simulink model "master_thesis_simulink"  (R2022a)
settings: Solver=VariableStepAuto  StartTime=0.0  StopTime=p_0p.time(end)  FixedStep=0.001  RelTol=1e-3
values from neighbouring files (symbols this model uses):
  markers_forearm = [0.00210510253906 -0.143263397217 -0.00798474121094]    [markers_forearm.mat]
  markers_shoulder = [0.010127746582 -0.151647644043 -0.0119686279297]    [markers_shoulder.mat]
undefined symbols (not defined in the file or in its folder): arm, DiscIntNeverNeededParam, Discrete, ekf, kf, LS, m, markers_hand, n, noise, q0, q0_LS, q0_model, sample_Time, selected, state_observer, Time, tSh_0_0Conf, X, Y, Z
libraries: sm_lib x2029, nesl_utility x1553, robotlib x75, ctrlSharedLib x8
(part 68 of 70)

== matlab function master_thesis_simulink/Ros2Matlab/S1_F0_H3/Position_M0 & velocity_M0 computation/MATLAB Function3 ==
  data: M0_isNew input; y output; M1_isNew input; M2_isNew input; M3_isNew input; M4_isNew input
 function y = fcn(M0_isNew, M1_isNew, M2_isNew, M3_isNew, M4_isNew)

if (M0_isNew == 0 || M1_isNew == 0 || M2_isNew == 0 || M3_isNew == 0 || M4_isNew == 0)
%if (M0_isNew == 0 || M1_isNew == 0 || M2_isNew == 0)

    y = -1;

else

    y = 1;
end

== matlab function master_thesis_simulink/Ros2Matlab/S1_F0_H3/tSh_0 computation/If Action Subsystem1/Mi_M0_POS1 ==
  data: p0_W input; pSh_W input; quat_02W input; tSh_0 output
function tSh_0  = fcn(p0_W, pSh_W, quat_02W)

% p_0 and v_0 are wrt M0_RF
% p_Sh wrt Sh_RF
% p_Fo wrt Fo_RF
% p_Wr wrt Wr_RF

% Number of markers
%m = size(p_W, 1) / 3;

%% Position/velocity of the markers wrt M0
tSh_0 = zeros(3, 1);

%% Quaternion describing rotation of M0 wrt W
quat_02W = reshape(quat_02W(1:4), [1, 4]);

%R =Rz*Ry*Rx;

%% Rotation: 0 to W
R_02W = quat2rotm(quat_02W);


tSh_0 = -R_02W'*p0_W + R_02W'*pSh_W;

== matlab function master_thesis_simulink/Ros2Matlab/S1_F0_H3/tSh_0 computation/MATLAB Function3 ==
  data: M0_isNew input; y output; Sh_isNew input
function y = fcn(M0_isNew, Sh_isNew)

if (M0_isNew == 0 || Sh_isNew == 0)

    y = -1;

else

    y = 1;
end

== matlab function master_thesis_simulink/Experiments/S1_F0_H3/Experiments/EKF/Extended Kalman Filter ==
  settings: updateMethod=DISCRETE
  data: p_0p input; v_0p input; shoulder_variables input; forearm_variables input; hand_variables input; qk output; Pk output; ekf parameter; noise parameter
function [qk, Pk] = KF(p_0p, v_0p, shoulder_variables, forearm_variables, hand_variables, ekf, noise)

% Extended Kalman filter algorithm 
% The following EKF algorithm estimate the state qk based on :
% -- The previous estimate qk_1 
% -- The input v_0 at time k
% -- The measurement p_0 at time k

% Inputs:
% -- p_0        : Measurement at time k
% -- v_0        : Input at time k

% Output:
% -- qk         : EKF estimate 
% -- Pk         : Covariance matrix of the state

%% Extrinsic functions
coder.extrinsic('f_f_mex');
coder.extrinsic('f_Phi_mex');
coder.extrinsic('f_Fekf_mex');
coder.extrinsic('f_Gekf_mex');
coder.extrinsic('f_Hekf_mex');
coder.extrinsic('eigs');

%% Define flags to understand if there are any markers in SHOULDER, FOREARM, HAND
flag_sh = shoulder_variables;
flag_fo = forearm_variables;
flag_ha = hand_variables;

if (shoulder_variables == -1)

    flag_sh = [];
end

if (forearm_variables == -1)

    flag_fo = [];
end

if (hand_variables == -1)

    flag_ha = [];
end

%% Number of markers
m = size(p_0p, 1) / 3;

%% Number of DoF
n = size(ekf.q0, 1);

%% Initialization

% Fk initialization
Fk = zeros(n, n);

% Gk initialization
Gk = zeros(n, m*3);

% Hk initialization
Hk = zeros(m*3, n);

% Phi_qk_ initialization
Phi_qk_ = zeros(m*3, 1);

% qk_ initialization
qk_ = zeros(n, 1);

%% Current state estimate, covariance
persistent qk_1 Pk_1;

if isempty(qk_1)

    %% %% First iteration
    qk = ekf.q0;
    qk_1 = qk;
    Pk = ekf.P0;
    Pk_1 = Pk;

else
   
    %% %% Next iterations

    %% Process Noise 
    % Gk computation
    Gk = full(f_Gekf_mex(qk_1, flag_sh, flag_fo, flag_ha, v_0p));

    % Q
%     noise.Q = Gk * noise.Rv * Gk'* 100;
%     noise.Q = (noise.Q + noise.Q') / 2; 
%     
%     % Check if Q is a Covariance matrix
%     is_Symmetric = issymmetric(noise.Q);
%     is_PosDef = false;
%     if ~is_Symmetric
% 
%         disp('Q not Symmetric');
%     else
%         
%         eig = zeros(n, 1);
%         eig = eigs(noise.Q, n);
%         if all(eig > 0)
%             is_PosDef = true;
%         end
%     end
% 
%     if ~is_PosDef
% 
%         disp('Q not Positve Definite');       
%     end
    
    %% TIME update
    % Predicted state
    qk_ = full(f_f_mex(qk_1, flag_sh, flag_fo, flag_ha, v_0p));

    % Fk computation
    Fk = full(f_Fekf_mex(qk_1, flag_sh, flag_fo, flag_ha, v_0p));

    % Predicted Covariance
    Pk_ = Fk * Pk_1 * Fk' + noise.Q;
    
    %% MEASUREMENT update
    % Hk computation
    Hk = full(f_Hekf_mex(qk_, flag_sh, flag_fo, flag_ha));

    % Kalman Gain 
    Kk = Pk_ * Hk' / (Hk * Pk_ * Hk' + noise.R);

    % Phi(qk_)
    Phi_qk_ = full(f_Phi_mex(qk_, flag_sh, flag_fo, flag_ha));

    % Updated state
    qk = wrapToPi(qk_ + Kk * (p_0p - Phi_qk_));
    qk_1 = qk;

    % Updated Covariance
    Pk = (eye(n) - Kk * Hk) * Pk_ * (eye(n) - Kk * Hk)' + Kk * noise.R * Kk';
    Pk_1 = Pk;

end
end

== matlab function master_thesis_simulink/Experiments/S1_F0_H3/Experiments/EKF/p_0p - Phi(q_EKF) ==
  data: p_0p input; q_EKF input; error_FK output; shoulder_variables input; forearm_variables input; hand_variables input
function error_FK  = FK(p_0p, q_EKF, shoulder_variables, forearm_variables, hand_variables)

% Computes the joints' velocities (LEAST SQUARES)

% Inputs:
% -- q                     : current joint variables configuration
% -- u                     : markers' velocities measurements
% -- shoulder_variables    : matrix containing markers position wrt SHOULDER Base RF
% -- forearm_variables     : matrix containing markers position wrt FOREARM Base RF
% -- hand_variables        : matrix containing markers position wrt HAND Base RF


% Output:
% -- Phi                   : Position of the markers wrt World RF
% -- J                     : Jacobian evaluated at the current joints variables estimate

% Extrinsic functions
coder.extrinsic('f_Phi_mex');
 
% Define flags to understand if there are any markers in SHOULDER, FOREARM, HAND
flag_sh = shoulder_variables;
flag_fo = forearm_variables;
flag_ha = hand_variables;

if (shoulder_variables == -1)

    flag_sh = [];
end

if (forearm_variables == -1)

    flag_fo = [];
end

if (hand_variables == -1)

    flag_ha = [];
end

% Initialization
p_FK = zeros(12, 1);

% Phi(q_EKF)
p_FK = full(f_Phi_mex(q_EKF, flag_sh, flag_fo, flag_ha));

% p_0 - Phi(q_EKF)
error_FK = p_0p - p_FK;

== matlab function master_thesis_simulink/Experiments/S1_F0_H3/Experiments/Human arm/MATLAB Function2 ==
  data: shoulder input; y output
function y = fcn(shoulder)

y = shoulder(1:3, :);

== matlab function master_thesis_simulink/Experiments/S1_F0_H3/Experiments/Human arm/MATLAB Function3 ==
  data: forearm input; y output
function y = fcn(forearm)

y = forearm(1:3, :);

== matlab function master_thesis_simulink/Experiments/S1_F0_H3/Experiments/Human arm/MATLAB Function4 ==
  data: hand input; y output size=[3 2]
function y = fcn(hand)

y = hand(1:3, :);

== matlab function master_thesis_simulink/Experiments/S1_F0_H3/Experiments/KF/Kalman Filter ==
  data: Delta_pk input; Delta_uk input; Delta_qk output; kf parameter; Pk output; noise parameter; p00 input
function [Delta_qk, Pk] = KF(Delta_pk, Delta_uk, kf, noise, p00)

% Kalman filter algorithm 
% The following KF algorithm estimate the quantity Delta_qk based on :
% -- The previous estimate xk_1 
% -- The input u_eqk at time k
% -- The measurement Delta_pk at time k

% Inputs:
% -- Delta_pk       : Measurement at time k
% -- Delta_uk       : Input at time k

% Output:
% -- Delta_qk       : KF estimate 
% -- Pk             : Covariance matrix of the state

persistent iteration;
% Previous state estimate
persistent Delta_qk_1 Pk_1;

persistent Delta_pk_1 Delta_uk_1

% Number of markers
m = size(kf.H, 1) / 3;
% Number of DoF
n = size(kf.F, 1);

% qk_ initialization
Delta_qk_ = zeros(n, 1);

% qk initialization
Delta_qk = zeros(n, 1);

% Pk initialization
Pk = zeros(n, n);

% Initialization
% if isempty(iteration)
% 
%     iteration = 1;
%     Delta_qk_1 = kf.Delta_q0;
%     Delta_qk = Delta_qk_1;
%     Pk = kf.Pk(1:n, 1:n);
%     iteration = iteration + 1;
% 
% else
% 
%     % Prediction ste
%     Delta_qk_ = kf.F * Delta_qk_1 + kf.G * u_eq;
%     
%     % Update step
%     Delta_qk = Delta_qk_ + kf.Kk(1:n, 3*m*(iteration-2)+1:3*m*(iteration-2)+3*m) * (Delta_pk - kf.H * Delta_qk_);
% 
%     if (iteration < 10)
% 
%         disp(abs(Delta_qk - Delta_qk_1))
%     end
%     Delta_qk_1 = Delta_qk;
%     Pk = kf.Pk(1:n, n*(iteration-1)+1:n*(iteration-1)+n);
%     iteration = iteration + 1;
% end

if isempty(Delta_qk_1)

    iteration = 1;

 
    % MEASUREMENT update
    Kk = p00 * kf.H' / (kf.H * p00 * kf.H' + noise.R);
    Delta_qk = Kk * (Delta_pk - kf.H*kf.Delta_q0);
    Delta_qk_1 = Delta_qk;
    Pk = p00;
    Pk_1 = Pk;
else
    
    % TIME update
    Delta_qk_ = kf.F*Delta_qk_1 + kf.G*Delta_uk;
    Pk_ = kf.F * Pk_1 * kf.F' + noise.Q;
    
    % MEASUREMENT update
    Kk = Pk_ * kf.H' / (kf.H * Pk_ * kf.H' + noise.R);
    Delta_qk = Delta_qk_ + Kk * (Delta_pk - kf.H*Delta_qk_);
    
    Delta_qk_1 = Delta_qk;
    Pk = (eye(n) - Kk * kf.H) * Pk_ * (eye(n) - Kk * kf.H)' + Kk * noise.R * Kk';
    Pk_1 = Pk;
    
    if (iteration == 2)
    
        disp('KF ')
        disp(Kk);
    end
end

iteration = iteration + 1;
end

== matlab function master_thesis_simulink/Experiments/S1_F0_H3/Experiments/KF/MATLAB Function ==
  data: n_k output; noise parameter
function n_k = fcn(noise)

% Generate a sample from normal distribution with covariance matrix N
coder.extrinsic('mvnrnd');

% Number of markers 
m = size(noise.N, 1) / 3;

% Initialization
n_k = zeros(m*3, 1);

n_k = mvnrnd(zeros(m*3, 1), noise.N, 1)';

== matlab function master_thesis_simulink/Experiments/S1_F0_H3/Experiments/KF/trial/Kalman Filter ==
  data: Delta_pk input; Delta_uk input; Delta_qk output; kf parameter; Pk output
function [Delta_qk, Pk] = KF(Delta_pk, Delta_uk, kf)

% Kalman filter algorithm 
% The following KF algorithm estimate the quantity Delta_qk based on :
% -- The previous estimate xk_1 
% -- The input u_eqk at time k
% -- The measurement Delta_pk at time k

% Inputs:
% -- Delta_pk       : Measurement at time k
% -- Delta_uk       : Input at time k

% Output:
% -- Delta_qk       : KF estimate 
% -- Pk             : Covariance matrix of the state

persistent iteration;
% Previous state estimate
persistent Delta_qk_1;

% Number of markers
m = size(kf.H, 1) / 3;
% Number of DoF
n = size(kf.F, 1);

% Initialization
if isempty(iteration)

    iteration = 1;
    Delta_qk_1 = kf.x0est;
    Delta_qk = Delta_qk_1;
    Pk = kf.Pk(1:n, 1:n);
    iteration = iteration + 1;

else

    % Prediction step
    Delta_qk_ = kf.F * Delta_qk_1 - kf.G * Delta_uk;
    
    % Update step
    Delta_qk = Delta_qk_ + kf.Kk(1:n, 3*m*(iteration-2)+1:3*m*(iteration-2)+3*m) * (Delta_pk - kf.H * Delta_qk_);
    Delta_qk_1 = Delta_qk;
    Pk = kf.Pk(1:n, n*(iteration-1)+1:n*(iteration-1)+n);
    iteration = iteration + 1;
end

== matlab function master_thesis_simulink/Experiments/S1_F1_H2/Experiments/EKF/Extended Kalman Filter ==
  settings: updateMethod=DISCRETE
  data: p_0p input; v_0p input; shoulder_variables input; forearm_variables input; hand_variables input; qk output; Pk output; ekf parameter; noise parameter
function [qk, Pk] = KF(p_0p, v_0p, shoulder_variables, forearm_variables, hand_variables, ekf, noise)

% Extended Kalman filter algorithm 
% The following EKF algorithm estimate the state qk based on :
% -- The previous estimate qk_1 
% -- The input v_0 at time k
% -- The measurement p_0 at time k

% Inputs:
% -- p_0        : Measurement at time k
% -- v_0        : Input at time k

% Output:
% -- qk         : EKF estimate 
% -- Pk         : Covariance matrix of the state

%% Extrinsic functions
coder.extrinsic('f_f_mex');
coder.extrinsic('f_Phi_mex');
coder.extrinsic('f_Fekf_mex');
coder.extrinsic('f_Gekf_mex');
coder.extrinsic('f_Hekf_mex');
coder.extrinsic('eigs');

%% Define flags to understand if there are any markers in SHOULDER, FOREARM, HAND
flag_sh = shoulder_variables;
flag_fo = forearm_variables;
flag_ha = hand_variables;

if (shoulder_variables == -1)

    flag_sh = [];
end

if (forearm_variables == -1)

    flag_fo = [];
end

if (hand_variables == -1)

    flag_ha = [];
end

%% Number of markers
m = size(p_0p, 1) / 3;

%% Number of DoF
n = size(ekf.q0, 1);

%% Initialization

% Fk initialization
Fk = zeros(n, n);

% Gk initialization
Gk = zeros(n, m*3);

% Hk initialization
Hk = zeros(m*3, n);

% Phi_qk_ initialization
Phi_qk_ = zeros(m*3, 1);

% qk_ initialization
qk_ = zeros(n, 1);

%% Current state estimate, covariance
persistent qk_1 Pk_1;

if isempty(qk_1)

    %% %% First iteration
    qk = ekf.q0;
    qk_1 = qk;
    Pk = ekf.P0;
    Pk_1 = Pk;

else
   
    %% %% Next iterations

    %% Process Noise 
    % Gk computation
    Gk = full(f_Gekf_mex(qk_1, flag_sh, flag_fo, flag_ha, v_0p));

    % Q
%     noise.Q = Gk * noise.Rv * Gk'* 100;
%     noise.Q = (noise.Q + noise.Q') / 2; 
%     
%     % Check if Q is a Covariance matrix
%     is_Symmetric = issymmetric(noise.Q);
%     is_PosDef = false;
%     if ~is_Symmetric
% 
%         disp('Q not Symmetric');
%     else
%         
%         eig = zeros(n, 1);
%         eig = eigs(noise.Q, n);
%         if all(eig > 0)
%             is_PosDef = true;
%         end
%     end
% 
%     if ~is_PosDef
% 
%         disp('Q not Positve Definite');       
%     end
    
    %% TIME update
    % Predicted state
    qk_ = full(f_f_mex(qk_1, flag_sh, flag_fo, flag_ha, v_0p));

    % Fk computation
    Fk = full(f_Fekf_mex(qk_1, flag_sh, flag_fo, flag_ha, v_0p));

    % Predicted Covariance
    Pk_ = Fk * Pk_1 * Fk' + noise.Q;
    
    %% MEASUREMENT update
    % Hk computation
    Hk = full(f_Hekf_mex(qk_, flag_sh, flag_fo, flag_ha));

    % Kalman Gain 
    Kk = Pk_ * Hk' / (Hk * Pk_ * Hk' + noise.R);

    % Phi(qk_)
    Phi_qk_ = full(f_Phi_mex(qk_, flag_sh, flag_fo, flag_ha));

    % Updated state
    qk = wrapToPi(qk_ + Kk * (p_0p - Phi_qk_));
    qk_1 = qk;

    % Updated Covariance
    Pk = (eye(n) - Kk * Hk) * Pk_ * (eye(n) - Kk * Hk)' + Kk * noise.R * Kk';
    Pk_1 = Pk;

end
end

== matlab function master_thesis_simulink/Experiments/S1_F0_H3/Experiments/KF/trial/Linearized Discrete Model ==
  data: Delta_uk input; Delta_qk output; Delta_pk output; kf parameter
function [Delta_qk, Delta_pk] = LDM(Delta_uk, kf)

% Discrete model linearized around the equilibrium point [q_eq, u_eq]

% This function computes both the outputs (markers' position) and the
% states (joints' variables) without considering the measurement noise

% Delta_qk+1 = F*Delta_qk + G*Delta_uk
% Delta_pk = H*Delta_qk

% Input:
% -- Delta_uk       : Delta_uk = uk - u_eqk at time k

% Output:
% -- Delta_qk       : States at time k
% -- Delta_pk       : outputs at time k

% Previous state
persistent Delta_qk_1; 

if isempty(Delta_qk_1)

    % Initial condition
    Delta_qk_1 = kf.q0 - kf.equilibrium_q;
    Delta_qk = Delta_qk_1;

else

    % State equation
    Delta_qk = kf.F * Delta_qk_1 + kf.G * Delta_uk;
    Delta_qk_1 = Delta_qk;

end

% Output equation
Delta_pk = kf.H * Delta_qk;

== matlab function master_thesis_simulink/Experiments/S1_F0_H3/Experiments/LS/LS ==
  data: q input; v_0 input; qdot_LS output; shoulder_variables input; forearm_variables input; hand_variables input
function qdot_LS  = LS(q, v_0, shoulder_variables, forearm_variables, hand_variables)

% Computes the joints' velocities (LEAST SQUARES)

% Inputs:
% -- q                     : current joint variables configuration
% -- u                     : markers' velocities measurements
% -- shoulder_variables    : matrix containing markers position wrt SHOULDER Base RF
% -- forearm_variables     : matrix containing markers position wrt FOREARM Base RF
% -- hand_variables        : matrix containing markers position wrt HAND Base RF


% Output:
% -- Phi                   : Position of the markers wrt World RF
% -- J                     : Jacobian evaluated at the current joints variables estimate

% Extrinsic functions
coder.extrinsic('f_Jpseudo_exp_mex');
 
% Define flags to understand if there are any markers in SHOULDER, FOREARM, HAND
flag_sh = shoulder_variables;
flag_fo = forearm_variables;
flag_ha = hand_variables;

if (shoulder_variables == -1)

    flag_sh = [];
end

if (forearm_variables == -1)

    flag_fo = [];
end

if (hand_variables == -1)

    flag_ha = [];
end

% Number of joints
n = size(q, 1);

% Initialization
qdot_LS = zeros(n, 1);
J = zeros(12,7);

% Jacobian
%J = full(f_J_exp_mex('f_J_exp', q, flag_sh, flag_fo, flag_ha));
% Jpseudo = (J'*J)^(-1)*J';

Jpseudo = full(f_Jpseudo_exp_mex('f_Jpseudo_exp', q, flag_sh, flag_fo, flag_ha));

qdot_LS = Jpseudo * v_0;

== matlab function master_thesis_simulink/Experiments/S1_F0_H3/Experiments/LS/p_0 - Phi(q_LS) ==
  data: p_0 input; q_LS input; error_FK output; shoulder_variables input; forearm_variables input; hand_variables input
function error_FK  = LS(p_0, q_LS, shoulder_variables, forearm_variables, hand_variables)

% Computes the joints' velocities (LEAST SQUARES)

% Inputs:
% -- q                     : current joint variables configuration
% -- u                     : markers' velocities measurements
% -- shoulder_variables    : matrix containing markers position wrt SHOULDER Base RF
% -- forearm_variables     : matrix containing markers position wrt FOREARM Base RF
% -- hand_variables        : matrix containing markers position wrt HAND Base RF


% Output:
% -- Phi                   : Position of the markers wrt World RF
% -- J                     : Jacobian evaluated at the current joints variables estimate

% Extrinsic functions
coder.extrinsic('f_Phi_exp_mex');
 
% Define flags to understand if there are any markers in SHOULDER, FOREARM, HAND
flag_sh = shoulder_variables;
flag_fo = forearm_variables;
flag_ha = hand_variables;

if (shoulder_variables == -1)

    flag_sh = [];
end

if (forearm_variables == -1)

    flag_fo = [];
end

if (hand_variables == -1)

    flag_ha = [];
end

% Initialization
p_FK = zeros(12, 1);

% Phi(q_EKF)
p_FK = full(f_Phi_exp_mex(q_LS, flag_sh, flag_fo, flag_ha));

% p_0 - Phi(q_EKF)
error_FK = p_0 - p_FK;

== matlab function master_thesis_simulink/Experiments/S1_F0_H3/MATLAB Function3 ==
  data: isNew input; y output
 function y = fcn(isNew)

if (isNew == -1)

    y = -1;

else

    y = 1;
end

== matlab function master_thesis_simulink/Experiments/S1_F0_H3/Model validation/Average ==
  data: pk input; pk_hat output
function pk_hat = fcn(pk)

persistent k pk_1_hat;

if isempty(k)

    k = 1;
    pk_hat = pk;
    pk_1_hat = pk_hat;

else

    k = k + 1;
    pk_hat = pk_1_hat + 1/k * (pk - pk_1_hat);
    pk_1_hat = pk_hat;
end

== matlab function master_thesis_simulink/Experiments/S1_F0_H3/Model validation/Markers_Bases ==
  data: p_0p_mean input; markers_shoulder output; arm parameter; markers_forearm output; markers_hand output
function [markers_shoulder, markers_forearm, markers_hand] = fcn(p_0p_mean, arm)

m = size(p_0p_mean, 1) / 3;

markers_shoulder = zeros(3, 1);
markers_forearm = -1;
markers_hand = zeros(3, 3);

 
for i = 1 : m

    % Shoulder
    if (i == 1)

        markers_shoulder = p_0p_mean(1:3);
    
    % Hand
    elseif (i > 1)

        markers_hand(:, i-1) = p_0p_mean((i-1)*3+1:(i-1)*3+3);
        markers_hand(2, i-1) = markers_hand(2, i-1) + arm.shoulder.length + arm.forearm.length;
    end

end

== matlab function master_thesis_simulink/Experiments/S1_F0_H3/Model validation/p_v__vs_FK_J ==
  data: q input; p_Model output; shoulder_variables input; forearm_variables input; hand_variables input
function p_Model  = FK_J(q, shoulder_variables, forearm_variables, hand_variables)

% Computes the joints' velocities (LEAST SQUARES)

% Inputs:
% -- q                     : current joint variables configuration
% -- u                     : markers' velocities measurements
% -- shoulder_variables    : matrix containing markers position wrt SHOULDER Base RF
% -- forearm_variables     : matrix containing markers position wrt FOREARM Base RF
% -- hand_variables        : matrix containing markers position wrt HAND Base RF


% Output:
% -- Phi                   : Position of the markers wrt World RF

% Extrinsic functions
coder.extrinsic('f_Phi_mex');
 
% Define flags to understand if there are any markers in SHOULDER, FOREARM, HAND
flag_sh = shoulder_variables;
flag_fo = forearm_variables;
flag_ha = hand_variables;

if (shoulder_variables == -1)

    flag_sh = [];
end

if (forearm_variables == -1)

    flag_fo = [];
end

if (hand_variables == -1)

    flag_ha = [];
end

% Initialization
p_Model = zeros(12, 1);

% FK
p_Model = full(f_Phi_mex(q, flag_sh, flag_fo, flag_ha));

== matlab function master_thesis_simulink/Experiments/S1_F0_H3/Noise estimation/Average ==
  data: Rp0_W input; Rpi_W input; Rpi_0p output; Rv0_W input; Rvi_W input; Rvi_0p output
function [Rpi_0p, Rvi_0p] = fcn(Rp0_W, Rpi_W, Rv0_W, Rvi_W)

coder.extrinsic('format');
format longE;

% Number of markers
m = size(Rpi_W, 1) / 3; 

%% Rotation of pi/2 along z
Rzpi2 = [0 -1 0;
         1 0 0;
         0 0 1];

%% Covariance Noise of pi^0'
Rpi_0p = zeros(3*m, 3);

for i = 1:m

        Rpi_0p(1+(i-1)*3:3+(i-1)*3, :) = Rzpi2 * (Rp0_W + Rpi_W(1+(i-1)*3:3+(i-1)*3, :)) * Rzpi2';
        Rpi_0p(1+(i-1)*3:3+(i-1)*3, :) = (Rpi_0p(1+(i-1)*3:3+(i-1)*3, :) + Rpi_0p(1+(i-1)*3:3+(i-1)*3, :)') / 2;
end

%% Covariance Noise of vi^0
Rvi_0p = zeros(3*m, 3);

for i = 1:m

        Rvi_0p(1+(i-1)*3:3+(i-1)*3, :) = Rzpi2 * (Rv0_W + Rvi_W(1+(i-1)*3:3+(i-1)*3, :)) * Rzpi2';
        Rvi_0p(1+(i-1)*3:3+(i-1)*3, :) = (Rvi_0p(1+(i-1)*3:3+(i-1)*3, :) + Rvi_0p(1+(i-1)*3:3+(i-1)*3, :)') / 2;
end

== matlab function master_thesis_simulink/Experiments/S1_F0_H3/Noise estimation/Noise Covariance of pi_0 Average ==
  data: Rk input; Rk_hat output
function Rk_hat= fcn(Rk)

persistent k Rk_1_hat;

if isempty(k)

    k = 1;
    Rk_hat = Rk;
    Rk_1_hat = Rk_hat;

else

    k = k + 1;
    Rk_hat = Rk_1_hat + 1/k * (Rk - Rk_1_hat);
    Rk_1_hat = Rk_hat;
end

== matlab function master_thesis_simulink/Experiments/S1_F0_H3/Noise estimation/Noise Covariance of vi_0 Average ==
  data: Rk input; Rk_hat output
function Rk_hat= fcn(Rk)

persistent k Rk_1_hat;

if isempty(k)

    k = 1;
    Rk_hat = Rk;
    Rk_1_hat = Rk_hat;

else

    k = k + 1;
    Rk_hat = Rk_1_hat + 1/k * (Rk - Rk_1_hat);
    Rk_1_hat = Rk_hat;
end

== matlab function master_thesis_simulink/Ros2Matlab/S1_F2_H2/Position_M0 & velocity_M0 computation/ /Mi_M0_POS ==
  data: p_W input; v_W input; quat_02W input; p_0p output; v_0p output
function [p_0p , v_0p] = fcn(p_W, v_W, quat_02W)

% p_0 and v_0 are wrt M0_RF
% p_0p and v_0p are wrt M0'_RF

% Number of markers
m = size(p_W, 1) / 3 - 1; 

%% Position/velocity of the markers wrt M0
p_0 = zeros(3*m, 1);
v_0 = zeros(3*m, 1);

%% Position/velocity of the markers wrt M0'
p_0p = zeros(3*m, 1);
v_0p = zeros(3*m, 1);

%% Quaternion describing rotation of M0 wrt W
quat_02W = reshape(quat_02W(1:4), [1, 4]);

%% Rotation: 0 to W
Rot_02W = quat2rotm(quat_02W);

%% Rotation of pi/2 along z
Rzpi2 = [0 -1 0;
         1 0 0;
         0 0 1];
%% Position/velocity of 0 wrt W
p0_W = p_W(1:3);
v0_W = v_W(1:3);

%% Position of markers wrt 0'
for i = 1:m

        p_0(1+(i-1)*3:3+(i-1)*3) = -Rot_02W' * p0_W + Rot_02W' * p_W(1+(i)*3:3+(i)*3);
        p_0p(1+(i-1)*3:3+(i-1)*3) = Rzpi2 * Rot_02W * p_0(1+(i-1)*3:3+(i-1)*3);
        v_0(1+(i-1)*3:3+(i-1)*3) = -Rot_02W'*v0_W + Rot_02W'*v_W(1+(i)*3:3+(i)*3);
        v_0p(1+(i-1)*3:3+(i-1)*3) = Rzpi2 * Rot_02W * v_0(1+(i-1)*3:3+(i-1)*3);
end

== matlab function master_thesis_simulink/Ros2Matlab/S1_F2_H2/Position_M0 & velocity_M0 computation/MATLAB Function3 ==
  data: M0_isNew input; y output; M1_isNew input; M2_isNew input; M3_isNew input; M4_isNew input; M5_isNew input
 function y = fcn(M0_isNew, M1_isNew, M2_isNew, M3_isNew, M4_isNew, M5_isNew)

if (M0_isNew == 0 || M1_isNew == 0 || M2_isNew == 0 || M3_isNew == 0 || M4_isNew == 0 || M5_isNew == 0)
%if (M0_isNew == 0 || M1_isNew == 0 || M2_isNew == 0)

    y = -1;

else

    y = 1;
end

== matlab function master_thesis_simulink/Ros2Matlab/S1_F2_H2/tSh_0 computation/If Action Subsystem1/Mi_M0_POS1 ==
  data: p0_W input; pSh_W input; quat_02W input; tSh_0 output
function tSh_0  = fcn(p0_W, pSh_W, quat_02W)

% p_0 and v_0 are wrt M0_RF
% p_Sh wrt Sh_RF
% p_Fo wrt Fo_RF
% p_Wr wrt Wr_RF

% Number of markers
%m = size(p_W, 1) / 3;

%% Position/velocity of the markers wrt M0
tSh_0 = zeros(3, 1);

%% Quaternion describing rotation of M0 wrt W
quat_02W = reshape(quat_02W(1:4), [1, 4]);

%R =Rz*Ry*Rx;

%% Rotation: 0 to W
R_02W = quat2rotm(quat_02W);


tSh_0 = -R_02W'*p0_W + R_02W'*pSh_W;

== matlab function master_thesis_simulink/Ros2Matlab/S1_F2_H2/tSh_0 computation/MATLAB Function3 ==
  data: M0_isNew input; y output; Sh_isNew input
function y = fcn(M0_isNew, Sh_isNew)

if (M0_isNew == 0 || Sh_isNew == 0)

    y = -1;

else

    y = 1;
end

== matlab function master_thesis_simulink/Experiments/S1_F2_H2/Experiments/EKF/Extended Kalman Filter ==
  settings: updateMethod=DISCRETE
  data: p_0p input; v_0p input; shoulder_variables input; forearm_variables input; hand_variables input; qk output; Pk output; ekf parameter; noise parameter
function [qk, Pk] = KF(p_0p, v_0p, shoulder_variables, forearm_variables, hand_variables, ekf, noise)

% Extended Kalman filter algorithm 
% The following EKF algorithm estimate the state qk based on :
% -- The previous estimate qk_1 
% -- The input v_0 at time k
% -- The measurement p_0 at time k

% Inputs:
% -- p_0        : Measurement at time k
% -- v_0        : Input at time k

% Output:
% -- qk         : EKF estimate 
% -- Pk         : Covariance matrix of the state

%% Extrinsic functions
coder.extrinsic('f_f_mex');
coder.extrinsic('f_Phi_mex');
coder.extrinsic('f_Fekf_mex');
coder.extrinsic('f_Gekf_mex');
coder.extrinsic('f_Hekf_mex');
coder.extrinsic('eigs');

%% Define flags to understand if there are any markers in SHOULDER, FOREARM, HAND
flag_sh = shoulder_variables;
flag_fo = forearm_variables;
flag_ha = hand_variables;

if (shoulder_variables == -1)

    flag_sh = [];
end

if (forearm_variables == -1)

    flag_fo = [];
end

if (hand_variables == -1)

    flag_ha = [];
end

%% Number of markers
m = size(p_0p, 1) / 3;

%% Number of DoF
n = size(ekf.q0, 1);

%% Initialization

% Fk initialization
Fk = zeros(n, n);

% Gk initialization
Gk = zeros(n, m*3);

% Hk initialization
Hk = zeros(m*3, n);

% Phi_qk_ initialization
Phi_qk_ = zeros(m*3, 1);

% qk_ initialization
qk_ = zeros(n, 1);

%% Current state estimate, covariance
persistent qk_1 Pk_1;

if isempty(qk_1)

    %% %% First iteration
    qk = ekf.q0;
    qk_1 = qk;
    Pk = ekf.P0;
    Pk_1 = Pk;

else
   
    %% %% Next iterations

    %% Process Noise 
    % Gk computation
    Gk = full(f_Gekf_mex(qk_1, flag_sh, flag_fo, flag_ha, v_0p));

    % Q
%     noise.Q = Gk * noise.Rv * Gk'* 100;
%     noise.Q = (noise.Q + noise.Q') / 2; 
%     
%     % Check if Q is a Covariance matrix
%     is_Symmetric = issymmetric(noise.Q);
%     is_PosDef = false;
%     if ~is_Symmetric
% 
%         disp('Q not Symmetric');
%     else
%         
%         eig = zeros(n, 1);
%         eig = eigs(noise.Q, n);
%         if all(eig > 0)
%             is_PosDef = true;
%         end
%     end
% 
%     if ~is_PosDef
% 
%         disp('Q not Positve Definite');       
%     end
    
    %% TIME update
    % Predicted state
    qk_ = full(f_f_mex(qk_1, flag_sh, flag_fo, flag_ha, v_0p));

    % Fk computation
    Fk = full(f_Fekf_mex(qk_1, flag_sh, flag_fo, flag_ha, v_0p));

    % Predicted Covariance
    Pk_ = Fk * Pk_1 * Fk' + noise.Q;
    
    %% MEASUREMENT update
    % Hk computation
    Hk = full(f_Hekf_mex(qk_, flag_sh, flag_fo, flag_ha));

    % Kalman Gain 
    Kk = Pk_ * Hk' / (Hk * Pk_ * Hk' + noise.R);

    % Phi(qk_)
    Phi_qk_ = full(f_Phi_mex(qk_, flag_sh, flag_fo, flag_ha));

    % Updated state
    qk = wrapToPi(qk_ + Kk * (p_0p - Phi_qk_));
    qk_1 = qk;

    % Updated Covariance
    Pk = (eye(n) - Kk * Hk) * Pk_ * (eye(n) - Kk * Hk)' + Kk * noise.R * Kk';
    Pk_1 = Pk;

end
end

== matlab function master_thesis_simulink/Experiments/S1_F1_H2/Noise estimation/Average ==
  data: Rp0_W input; Rpi_W input; Rpi_0p output; Rv0_W input; Rvi_W input; Rvi_0p output
function [Rpi_0p, Rvi_0p] = fcn(Rp0_W, Rpi_W, Rv0_W, Rvi_W)

coder.extrinsic('format');
format longE;

% Number of markers
m = size(Rpi_W, 1) / 3; 

%% Rotation of pi/2 along z
Rzpi2 = [0 -1 0;
         1 0 0;
         0 0 1];

%% Covariance Noise of pi^0'
Rpi_0p = zeros(3*m, 3);

for i = 1:m

        Rpi_0p(1+(i-1)*3:3+(i-1)*3, :) = Rzpi2 * (Rp0_W + Rpi_W(1+(i-1)*3:3+(i-1)*3, :)) * Rzpi2';
        Rpi_0p(1+(i-1)*3:3+(i-1)*3, :) = (Rpi_0p(1+(i-1)*3:3+(i-1)*3, :) + Rpi_0p(1+(i-1)*3:3+(i-1)*3, :)') / 2;
end

%% Covariance Noise of vi^0
Rvi_0p = zeros(3*m, 3);

for i = 1:m

        Rvi_0p(1+(i-1)*3:3+(i-1)*3, :) = Rzpi2 * (Rv0_W + Rvi_W(1+(i-1)*3:3+(i-1)*3, :)) * Rzpi2';
        Rvi_0p(1+(i-1)*3:3+(i-1)*3, :) = (Rvi_0p(1+(i-1)*3:3+(i-1)*3, :) + Rvi_0p(1+(i-1)*3:3+(i-1)*3, :)') / 2;
end

== matlab function master_thesis_simulink/Experiments/S1_F2_H2/Experiments/EKF/p_0p - Phi(q_EKF) ==
  data: p_0p input; q_EKF input; error_FK output; shoulder_variables input; forearm_variables input; hand_variables input
function error_FK  = FK(p_0p, q_EKF, shoulder_variables, forearm_variables, hand_variables)

% Computes the joints' velocities (LEAST SQUARES)

% Inputs:
% -- q                     : current joint variables configuration
% -- u                     : markers' velocities measurements
% -- shoulder_variables    : matrix containing markers position wrt SHOULDER Base RF
% -- forearm_variables     : matrix containing markers position wrt FOREARM Base RF
% -- hand_variables        : matrix containing markers position wrt HAND Base RF


% Output:
% -- Phi                   : Position of the markers wrt World RF
% -- J                     : Jacobian evaluated at the current joints variables estimate

% Extrinsic functions
coder.extrinsic('f_Phi_mex');
 
% Define flags to understand if there are any markers in SHOULDER, FOREARM, HAND
flag_sh = shoulder_variables;
flag_fo = forearm_variables;
flag_ha = hand_variables;

if (shoulder_variables == -1)

    flag_sh = [];
end

if (forearm_variables == -1)

    flag_fo = [];
end

if (hand_variables == -1)

    flag_ha = [];
end

% Initialization
p_FK = zeros(15, 1);

% Phi(q_EKF)
p_FK = full(f_Phi_mex(q_EKF, flag_sh, flag_fo, flag_ha));

% p_0 - Phi(q_EKF)
error_FK = p_0p - p_FK;

== matlab function master_thesis_simulink/Experiments/S1_F2_H2/Experiments/Human arm/MATLAB Function2 ==
  data: shoulder input; y output
function y = fcn(shoulder)

y = shoulder(1:3, :);

== matlab function master_thesis_simulink/Experiments/S1_F2_H2/Experiments/Human arm/MATLAB Function3 ==
  data: forearm input; y output
function y = fcn(forearm)

y = forearm(1:3, :);

== matlab function master_thesis_simulink/Experiments/S1_F2_H2/Experiments/Human arm/MATLAB Function4 ==
  data: hand input; y output size=[3 2]
function y = fcn(hand)

y = hand(1:3, :);

== matlab function master_thesis_simulink/Experiments/S1_F2_H2/Experiments/KF/Kalman Filter ==
  data: Delta_pk input; Delta_uk input; Delta_qk output; kf parameter; Pk output; noise parameter; p00 input
function [Delta_qk, Pk] = KF(Delta_pk, Delta_uk, kf, noise, p00)

% Kalman filter algorithm 
% The following KF algorithm estimate the quantity Delta_qk based on :
% -- The previous estimate xk_1 
% -- The input u_eqk at time k
% -- The measurement Delta_pk at time k

% Inputs:
% -- Delta_pk       : Measurement at time k
% -- Delta_uk       : Input at time k

% Output:
% -- Delta_qk       : KF estimate 
% -- Pk             : Covariance matrix of the state

persistent iteration;
% Previous state estimate
persistent Delta_qk_1 Pk_1;

persistent Delta_pk_1 Delta_uk_1

% Number of markers
m = size(kf.H, 1) / 3;
% Number of DoF
n = size(kf.F, 1);

% qk_ initialization
Delta_qk_ = zeros(n, 1);

% qk initialization
Delta_qk = zeros(n, 1);

% Pk initialization
Pk = zeros(n, n);

% Initialization
% if isempty(iteration)
% 
%     iteration = 1;
%     Delta_qk_1 = kf.Delta_q0;
%     Delta_qk = Delta_qk_1;
%     Pk = kf.Pk(1:n, 1:n);
%     iteration = iteration + 1;
% 
% else
% 
%     % Prediction ste
%     Delta_qk_ = kf.F * Delta_qk_1 + kf.G * u_eq;
%     
%     % Update step
%     Delta_qk = Delta_qk_ + kf.Kk(1:n, 3*m*(iteration-2)+1:3*m*(iteration-2)+3*m) * (Delta_pk - kf.H * Delta_qk_);
% 
%     if (iteration < 10)
% 
%         disp(abs(Delta_qk - Delta_qk_1))
%     end
%     Delta_qk_1 = Delta_qk;
%     Pk = kf.Pk(1:n, n*(iteration-1)+1:n*(iteration-1)+n);
%     iteration = iteration + 1;
% end

if isempty(Delta_qk_1)

    iteration = 1;

 
    % MEASUREMENT update
    Kk = p00 * kf.H' / (kf.H * p00 * kf.H' + noise.R);
    Delta_qk = Kk * (Delta_pk - kf.H*kf.Delta_q0);
    Delta_qk_1 = Delta_qk;
    Pk = p00;
    Pk_1 = Pk;
else
    
    % TIME update
    Delta_qk_ = kf.F*Delta_qk_1 + kf.G*Delta_uk;
    Pk_ = kf.F * Pk_1 * kf.F' + noise.Q;
    
    % MEASUREMENT update
    Kk = Pk_ * kf.H' / (kf.H * Pk_ * kf.H' + noise.R);
    Delta_qk = Delta_qk_ + Kk * (Delta_pk - kf.H*Delta_qk_);
    
    Delta_qk_1 = Delta_qk;
    Pk = (eye(n) - Kk * kf.H) * Pk_ * (eye(n) - Kk * kf.H)' + Kk * noise.R * Kk';
    Pk_1 = Pk;
    
    if (iteration == 2)
    
        disp('KF ')
        disp(Kk);
    end
end

iteration = iteration + 1;
end

== matlab function master_thesis_simulink/Experiments/S1_F2_H2/Experiments/KF/MATLAB Function ==
  data: n_k output; noise parameter
function n_k = fcn(noise)

% Generate a sample from normal distribution with covariance matrix N
coder.extrinsic('mvnrnd');

% Number of markers 
m = size(noise.N, 1) / 3;

% Initialization
n_k = zeros(m*3, 1);

n_k = mvnrnd(zeros(m*3, 1), noise.N, 1)';

== matlab function master_thesis_simulink/Experiments/S1_F2_H2/Experiments/KF/trial/Kalman Filter ==
  data: Delta_pk input; Delta_uk input; Delta_qk output; kf parameter; Pk output
function [Delta_qk, Pk] = KF(Delta_pk, Delta_uk, kf)

% Kalman filter algorithm 
% The following KF algorithm estimate the quantity Delta_qk based on :
% -- The previous estimate xk_1 
% -- The input u_eqk at time k
% -- The measurement Delta_pk at time k

% Inputs:
% -- Delta_pk       : Measurement at time k
% -- Delta_uk       : Input at time k

% Output:
% -- Delta_qk       : KF estimate 
% -- Pk             : Covariance matrix of the state

persistent iteration;
% Previous state estimate
persistent Delta_qk_1;

% Number of markers
m = size(kf.H, 1) / 3;
% Number of DoF
n = size(kf.F, 1);

% Initialization
if isempty(iteration)

    iteration = 1;
    Delta_qk_1 = kf.x0est;
    Delta_qk = Delta_qk_1;
    Pk = kf.Pk(1:n, 1:n);
    iteration = iteration + 1;

else

    % Prediction step
    Delta_qk_ = kf.F * Delta_qk_1 - kf.G * Delta_uk;
    
    % Update step
    Delta_qk = Delta_qk_ + kf.Kk(1:n, 3*m*(iteration-2)+1:3*m*(iteration-2)+3*m) * (Delta_pk - kf.H * Delta_qk_);
    Delta_qk_1 = Delta_qk;
    Pk = kf.Pk(1:n, n*(iteration-1)+1:n*(iteration-1)+n);
    iteration = iteration + 1;
end

== matlab function master_thesis_simulink/Experiments/S1_F2_H2/Experiments/KF/trial/Linearized Discrete Model ==
  data: Delta_uk input; Delta_qk output; Delta_pk output; kf parameter
function [Delta_qk, Delta_pk] = LDM(Delta_uk, kf)

% Discrete model linearized around the equilibrium point [q_eq, u_eq]

% This function computes both the outputs (markers' position) and the
% states (joints' variables) without considering the measurement noise

% Delta_qk+1 = F*Delta_qk + G*Delta_uk
% Delta_pk = H*Delta_qk

% Input:
% -- Delta_uk       : Delta_uk = uk - u_eqk at time k

% Output:
% -- Delta_qk       : States at time k
% -- Delta_pk       : outputs at time k

% Previous state
persistent Delta_qk_1; 

if isempty(Delta_qk_1)

    % Initial condition
    Delta_qk_1 = kf.q0 - kf.equilibrium_q;
    Delta_qk = Delta_qk_1;

else

    % State equation
    Delta_qk = kf.F * Delta_qk_1 + kf.G * Delta_uk;
    Delta_qk_1 = Delta_qk;

end

% Output equation
Delta_pk = kf.H * Delta_qk;

== matlab function master_thesis_simulink/Experiments/S1_F2_H2/Experiments/LS/LS ==
  data: q input; v_0 input; qdot_LS output; shoulder_variables input; forearm_variables input; hand_variables input
function qdot_LS  = LS(q, v_0, shoulder_variables, forearm_variables, hand_variables)

% Computes the joints' velocities (LEAST SQUARES)

% Inputs:
% -- q                     : current joint variables configuration
% -- u                     : markers' velocities measurements
% -- shoulder_variables    : matrix containing markers position wrt SHOULDER Base RF
% -- forearm_variables     : matrix containing markers position wrt FOREARM Base RF
% -- hand_variables        : matrix containing markers position wrt HAND Base RF


% Output:
% -- Phi                   : Position of the markers wrt World RF
% -- J                     : Jacobian evaluated at the current joints variables estimate

% Extrinsic functions
coder.extrinsic('f_Jpseudo_exp_mex');
 
% Define flags to understand if there are any markers in SHOULDER, FOREARM, HAND
flag_sh = shoulder_variables;
flag_fo = forearm_variables;
flag_ha = hand_variables;

if (shoulder_variables == -1)

    flag_sh = [];
end

if (forearm_variables == -1)

    flag_fo = [];
end

if (hand_variables == -1)

    flag_ha = [];
end

% Number of joints
n = size(q, 1);

% Initialization
qdot_LS = zeros(n, 1);
J = zeros(12,7);

% Jacobian
%J = full(f_J_exp_mex('f_J_exp', q, flag_sh, flag_fo, flag_ha));
% Jpseudo = (J'*J)^(-1)*J';

Jpseudo = full(f_Jpseudo_exp_mex('f_Jpseudo_exp', q, flag_sh, flag_fo, flag_ha));

qdot_LS = Jpseudo * v_0;

== matlab function master_thesis_simulink/Experiments/S1_F2_H2/Experiments/LS/p_0 - Phi(q_LS) ==
  data: p_0 input; q_LS input; error_FK output; shoulder_variables input; forearm_variables input; hand_variables input
function error_FK  = LS(p_0, q_LS, shoulder_variables, forearm_variables, hand_variables)

% Computes the joints' velocities (LEAST SQUARES)

% Inputs:
% -- q                     : current joint variables configuration
% -- u                     : markers' velocities measurements
% -- shoulder_variables    : matrix containing markers position wrt SHOULDER Base RF
% -- forearm_variables     : matrix containing markers position wrt FOREARM Base RF
% -- hand_variables        : matrix containing markers position wrt HAND Base RF


% Output:
% -- Phi                   : Position of the markers wrt World RF
% -- J                     : Jacobian evaluated at the current joints variables estimate

% Extrinsic functions
coder.extrinsic('f_Phi_exp_mex');
 
% Define flags to understand if there are any markers in SHOULDER, FOREARM, HAND
flag_sh = shoulder_variables;
flag_fo = forearm_variables;
flag_ha = hand_variables;

if (shoulder_variables == -1)

    flag_sh = [];
end

if (forearm_variables == -1)

    flag_fo = [];
end

if (hand_variables == -1)

    flag_ha = [];
end

% Initialization
p_FK = zeros(12, 1);

% Phi(q_EKF)
p_FK = full(f_Phi_exp_mex(q_LS, flag_sh, flag_fo, flag_ha));

% p_0 - Phi(q_EKF)
error_FK = p_0 - p_FK;

== matlab function master_thesis_simulink/Experiments/S1_F2_H2/MATLAB Function3 ==
  data: isNew input; y output
 function y = fcn(isNew)

if (isNew == -1)

    y = -1;

else

    y = 1;
end

== matlab function master_thesis_simulink/Experiments/S1_F2_H2/Model validation/Average ==
  data: pk input; pk_hat output
function pk_hat = fcn(pk)

persistent k pk_1_hat;

if isempty(k)

    k = 1;
    pk_hat = pk;
    pk_1_hat = pk_hat;

else

    k = k + 1;
    pk_hat = pk_1_hat + 1/k * (pk - pk_1_hat);
    pk_1_hat = pk_hat;
end

== matlab function master_thesis_simulink/System/Show Results/EKF/Phi(q_EKF) - p_0' ==
  data: q_EKF input; shoulder_variables input; forearm_variables input; hand_variables input; p_err output; p_0p input
function p_err   = Sing(q_EKF, shoulder_variables, forearm_variables, hand_variables, p_0p)

% Computes the joints' velocities (LEAST SQUARES)

% Inputs:
% -- q                     : current joint variables configuration
% -- u                     : markers' velocities measurements
% -- shoulder_variables    : matrix containing markers position wrt SHOULDER Base RF
% -- forearm_variables     : matrix containing markers position wrt FOREARM Base RF
% -- hand_variables        : matrix containing markers position wrt HAND Base RF


% Output:
% -- Phi                   : Position of the markers wrt World RF
% -- J                     : Jacobian evaluated at the current joints variables estimate

% Extrinsic functions
coder.extrinsic('f_Phi_mex');
coder.extrinsic('f_Fekf_mex');

% Define flags to understand if there are any markers in SHOULDER, FOREARM, HAND
flag_sh = shoulder_variables;
flag_fo = forearm_variables;
flag_ha = hand_variables;

if (shoulder_variables == -1)

    flag_sh = [];
end

if (forearm_variables == -1)

    flag_fo = [];
end

if (hand_variables == -1)

    flag_ha = [];
end

m = 0;
% S1_F1_H2
if (size(flag_sh, 2) == 1 && size(flag_fo, 2) == 1 && size(flag_ha, 2) == 2)

    % Number of markes
    m = 4;
 
% S0_F1_H2
elseif (size(flag_sh, 2) == 0 && size(flag_fo, 2) == 1 && size(flag_ha, 2) == 2)

    % Number of markes
    m = 3;
  
% S0_F2_H2
elseif (size(flag_sh, 2) == 0 && size(flag_fo, 2) == 2 && size(flag_ha, 2) == 2)

    % Number of markes
    m = 4;

% S1_F0_H2
elseif (size(flag_sh, 2) == 1 && size(flag_fo, 2) == 0 && size(flag_ha, 2) == 2)

    % Number of markes
    m = 3;

% S1_F0_H3
elseif (size(flag_sh, 2) == 1 && size(flag_fo, 2) == 0 && size(flag_ha, 2) == 3)

    % Number of markes
    m = 4;

% S1_F2_H2
elseif (size(flag_sh, 2) == 1 && size(flag_fo, 2) == 2 && size(flag_ha, 2) == 2)

    % Number of markes
    m = 5;

% S2_F0_H2
elseif(size(flag_sh, 2) == 2 && size(flag_fo, 2) == 0 && size(flag_ha, 2) == 2)

    % Number of markes
    m = 4; 
end

% Initialization
p = zeros(3*m, 1);

% Joints' velocities
p = full(f_Phi_mex(q_EKF, flag_sh, flag_fo, flag_ha));
p_err = p - p_0p;

== matlab function master_thesis_simulink/Experiments/S1_F2_H2/Model validation/Markers_Bases ==
  data: p_0p_mean input; markers_shoulder output; arm parameter; markers_forearm output; markers_hand output
function [markers_shoulder, markers_forearm, markers_hand] = fcn(p_0p_mean, arm)

m = size(p_0p_mean, 1) / 3;

markers_shoulder = zeros(3, 1);
markers_forearm = zeros(3, 2);
markers_hand = zeros(3, 2);

 
for i = 1 : m

    % Shoulder
    if (i == 1)

        markers_shoulder = p_0p_mean(1:3);

    % Forearm
    elseif (i == 2)

        markers_forearm(:, 1) = p_0p_mean(4:6);
        markers_forearm(2, 1) = markers_forearm(2, 1) + arm.shoulder.length;
     
       
   elseif (i == 3)

        markers_forearm(:, 2) = p_0p_mean(7:9);
        markers_forearm(2, 2) = markers_forearm(2, 2) + arm.shoulder.length;
    
    % Hand
    elseif (i > 3)

        markers_hand(:, i-3) = p_0p_mean((i-1)*3+1:(i-1)*3+3);
        markers_hand(2, i-3) = markers_hand(2, i-3) + arm.shoulder.length + arm.forearm.length;
    end

end

== matlab function master_thesis_simulink/Experiments/S1_F2_H2/Model validation/p_v__vs_FK_J ==
  data: q input; p_Model output; shoulder_variables input; forearm_variables input; hand_variables input
function p_Model  = FK_J(q, shoulder_variables, forearm_variables, hand_variables)

% Computes the joints' velocities (LEAST SQUARES)

% Inputs:
% -- q                     : current joint variables configuration
% -- u                     : markers' velocities measurements
% -- shoulder_variables    : matrix containing markers position wrt SHOULDER Base RF
% -- forearm_variables     : matrix containing markers position wrt FOREARM Base RF
% -- hand_variables        : matrix containing markers position wrt HAND Base RF


% Output:
% -- Phi                   : Position of the markers wrt World RF

% Extrinsic functions
coder.extrinsic('f_Phi_mex');
 
% Define flags to understand if there are any markers in SHOULDER, FOREARM, HAND
flag_sh = shoulder_variables;
flag_fo = forearm_variables;
flag_ha = hand_variables;

if (shoulder_variables == -1)

    flag_sh = [];
end

if (forearm_variables == -1)

    flag_fo = [];
end

if (hand_variables == -1)

    flag_ha = [];
end

% Number of markers
m = size(shoulder_variables, 2) + size(forearm_variables, 2) + size(hand_variables, 2);

% Initialization
p_Model = zeros(3*m, 1);

% FK
p_Model = full(f_Phi_mex(q, flag_sh, flag_fo, flag_ha));

== matlab function master_thesis_simulink/Experiments/S1_F2_H2/Noise estimation/Average ==
  data: Rp0_W input; Rpi_W input; Rpi_0p output; Rv0_W input; Rvi_W input; Rvi_0p output
function [Rpi_0p, Rvi_0p] = fcn(Rp0_W, Rpi_W, Rv0_W, Rvi_W)

coder.extrinsic('format');
format longE;

% Number of markers
m = size(Rpi_W, 1) / 3; 

%% Rotation of pi/2 along z
Rzpi2 = [0 -1 0;
         1 0 0;
         0 0 1];

%% Covariance Noise of pi^0'
Rpi_0p = zeros(3*m, 3);

for i = 1:m

        Rpi_0p(1+(i-1)*3:3+(i-1)*3, :) = Rzpi2 * (Rp0_W + Rpi_W(1+(i-1)*3:3+(i-1)*3, :)) * Rzpi2';
        Rpi_0p(1+(i-1)*3:3+(i-1)*3, :) = (Rpi_0p(1+(i-1)*3:3+(i-1)*3, :) + Rpi_0p(1+(i-1)*3:3+(i-1)*3, :)') / 2;
end

%% Covariance Noise of vi^0
Rvi_0p = zeros(3*m, 3);

for i = 1:m

        Rvi_0p(1+(i-1)*3:3+(i-1)*3, :) = Rzpi2 * (Rv0_W + Rvi_W(1+(i-1)*3:3+(i-1)*3, :)) * Rzpi2';
        Rvi_0p(1+(i-1)*3:3+(i-1)*3, :) = (Rvi_0p(1+(i-1)*3:3+(i-1)*3, :) + Rvi_0p(1+(i-1)*3:3+(i-1)*3, :)') / 2;
end

== matlab function master_thesis_simulink/Experiments/S1_F2_H2/Noise estimation/Noise Covariance of pi_0 Average ==
  data: Rk input; Rk_hat output
function Rk_hat= fcn(Rk)

persistent k Rk_1_hat;

if isempty(k)

    k = 1;
    Rk_hat = Rk;
    Rk_1_hat = Rk_hat;

else

    k = k + 1;
    Rk_hat = Rk_1_hat + 1/k * (Rk - Rk_1_hat);
    Rk_1_hat = Rk_hat;
end

== matlab function master_thesis_simulink/Experiments/S1_F2_H2/Noise estimation/Noise Covariance of vi_0 Average ==
  data: Rk input; Rk_hat output
function Rk_hat= fcn(Rk)

persistent k Rk_1_hat;

if isempty(k)

    k = 1;
    Rk_hat = Rk;
    Rk_1_hat = Rk_hat;

else

    k = k + 1;
    Rk_hat = Rk_1_hat + 1/k * (Rk - Rk_1_hat);
    Rk_1_hat = Rk_hat;
end

== matlab function master_thesis_simulink/System/Show Results/LS/Phi(q_LS) - p_0' ==
  data: q_LS input; shoulder_variables input; forearm_variables input; hand_variables input; p_err output; p_0p input
function p_err = Sing(q_LS, shoulder_variables, forearm_variables, hand_variables, p_0p)

% Computes the joints' velocities (LEAST SQUARES)

% Inputs:
% -- q                     : current joint variables configuration
% -- u                     : markers' velocities measurements
% -- shoulder_variables    : matrix containing markers position wrt SHOULDER Base RF
% -- forearm_variables     : matrix containing markers position wrt FOREARM Base RF
% -- hand_variables        : matrix containing markers position wrt HAND Base RF


% Output:
% -- Phi                   : Position of the markers wrt World RF
% -- J                     : Jacobian evaluated at the current joints variables estimate

% Extrinsic functions
coder.extrinsic('f_Phi_mex');

% Define flags to understand if there are any markers in SHOULDER, FOREARM, HAND
flag_sh = shoulder_variables;
flag_fo = forearm_variables;
flag_ha = hand_variables;

if (shoulder_variables == -1)

    flag_sh = [];
end

if (forearm_variables == -1)

    flag_fo = [];
end

if (hand_variables == -1)

    flag_ha = [];
end

m = 0;
% S1_F1_H2
if (size(flag_sh, 2) == 1 && size(flag_fo, 2) == 1 && size(flag_ha, 2) == 2)

    % Number of markes
    m = 4;
 
% S0_F1_H2
elseif (size(flag_sh, 2) == 0 && size(flag_fo, 2) == 1 && size(flag_ha, 2) == 2)

    % Number of markes
    m = 3;
  
% S0_F2_H2
elseif (size(flag_sh, 2) == 0 && size(flag_fo, 2) == 2 && size(flag_ha, 2) == 2)

    % Number of markes
    m = 4;

% S1_F0_H2
elseif (size(flag_sh, 2) == 1 && size(flag_fo, 2) == 0 && size(flag_ha, 2) == 2)

    % Number of markes
    m = 3;

% S1_F0_H3
elseif (size(flag_sh, 2) == 1 && size(flag_fo, 2) == 0 && size(flag_ha, 2) == 3)

    % Number of markes
    m = 4;

% S1_F2_H2
elseif (size(flag_sh, 2) == 1 && size(flag_fo, 2) == 2 && size(flag_ha, 2) == 2)

    % Number of markes
    m = 5;

% S2_F0_H2
elseif(size(flag_sh, 2) == 2 && size(flag_fo, 2) == 0 && size(flag_ha, 2) == 2)

    % Number of markes
    m = 4; 
end

% Initialization
p = zeros(3*m, 1);

% Joints' velocities
p = full(f_Phi_mex(q_LS, flag_sh, flag_fo, flag_ha));
p_err = p - p_0p;
